simulink model "ACC_ISO_test_001_cs"  (Simulink 7.6)
settings: Solver=ode5  SolverMode=SingleTasking  StartTime=0.0  StopTime=inf  FixedStep=1/100  RelTol=1e-3
PreLoadFcn:
  | check_NUTS_defined;
  | 
  | assignin('base',['model_closed_' bdroot],false);addpath('../includes_ACC');
InitFcn:
  | PreScanExperimentInitFcn(bdroot)
StopFcn:
  | PreScanExperimentStopFcn(bdroot)
undefined symbols (not defined in the file): DiscIntNeverNeededParam, x_ini_VRML, y_ini_VRML, z_ini_VRML
libraries: simulink x26, PreScanSimulinkLibrary x16, simulink_extras x9, PreScanUsefulBlocks x6, simulink_need_slupdate x1
(part 4 of 9)

== system ACC_ISO_test_001_cs/VISUWheels_Mazda_RX8_1 ==
  Wheels : Inport
  Demux : Demux  Outputs=[3 3 3 3 3 3 3 3]
  Saturation{,2,4,6} (4 alike) : Saturate  UpperLimit=[0.2 0.2 0.5]  LowerLimit=[-0.2 -0.2 -0.5]
  Saturation{1,3,5,8} (4 alike) : Saturate  UpperLimit=[30 inf 30]  LowerLimit=[-30 -inf -30]
  conv_RotWheelFL : Subsystem
  conv_RotWheelFR : Subsystem
  conv_RotWheelRL : Subsystem
  conv_RotWheelRR : Subsystem
  conv_TransWheelFL : Subsystem  mask(Translation node configuration){tp=Front-Left Wheel, gains=off, Gain_xISO=1, Gain_yISO=1, Gain_zISO=1}
      mask prompts: tp "Type"; gains "Edit scaling factors?"; Gain_xISO "Scaling factor in x-direction (ISO-convention)"; Gain_yISO "Scaling factor in y-direction (ISO-convention)"; Gain_zISO "Scaling factor in z-direction (ISO-convention)"
      mask init:
      | Visu_ini_param('Mazda_RX8',tp);
      mask StyleString: popup(Front-Left Wheel|Front-Right Wheel|Rear-Left Wheel|Rear-Right Wheel|Left Seat|Right Seat),checkbox,edit,edit,edit
      mask CallbackString:
      | |if strcmp(get_param(gcb, 'gains'),'on')
      |     set_param(gcb,'MaskVisibilities',{'on','on','on','on','on'})
      | else
      |     set_param(gcb,'MaskVisibilities',{'on','on','off','off','off'})
      | end|||
  conv_TransWheelFR : Subsystem  mask(Translation node configuration){tp=Front-Right Wheel, gains=off, Gain_xISO=1, Gain_yISO=1, Gain_zISO=1}
      mask prompts: tp "Type"; gains "Edit scaling factors?"; Gain_xISO "Scaling factor in x-direction (ISO-convention)"; Gain_yISO "Scaling factor in y-direction (ISO-convention)"; Gain_zISO "Scaling factor in z-direction (ISO-convention)"
      mask init:
      | Visu_ini_param('Mazda_RX8',tp);
      mask StyleString: popup(Front-Left Wheel|Front-Right Wheel|Rear-Left Wheel|Rear-Right Wheel|Left Seat|Right Seat),checkbox,edit,edit,edit
      mask CallbackString:
      | |if strcmp(get_param(gcb, 'gains'),'on')
      |     set_param(gcb,'MaskVisibilities',{'on','on','on','on','on'})
      | else
      |     set_param(gcb,'MaskVisibilities',{'on','on','off','off','off'})
      | end|||
  conv_TransWheelRL : Subsystem  mask(Translation node configuration){tp=Rear-Left Wheel, gains=off, Gain_xISO=1, Gain_yISO=1, Gain_zISO=1}
      mask prompts: tp "Type"; gains "Edit scaling factors?"; Gain_xISO "Scaling factor in x-direction (ISO-convention)"; Gain_yISO "Scaling factor in y-direction (ISO-convention)"; Gain_zISO "Scaling factor in z-direction (ISO-convention)"
      mask init:
      | Visu_ini_param('Mazda_RX8',tp);
      mask StyleString: popup(Front-Left Wheel|Front-Right Wheel|Rear-Left Wheel|Rear-Right Wheel|Left Seat|Right Seat),checkbox,edit,edit,edit
      mask CallbackString:
      | |if strcmp(get_param(gcb, 'gains'),'on')
      |     set_param(gcb,'MaskVisibilities',{'on','on','on','on','on'})
      | else
      |     set_param(gcb,'MaskVisibilities',{'on','on','off','off','off'})
      | end|||
  conv_TransWheelRR : Subsystem  mask(Translation node configuration){tp=Rear-Right Wheel, gains=off, Gain_xISO=1, Gain_yISO=1, Gain_zISO=1}
      mask prompts: tp "Type"; gains "Edit scaling factors?"; Gain_xISO "Scaling factor in x-direction (ISO-convention)"; Gain_yISO "Scaling factor in y-direction (ISO-convention)"; Gain_zISO "Scaling factor in z-direction (ISO-convention)"
      mask init:
      | Visu_ini_param('Mazda_RX8',tp);
      mask StyleString: popup(Front-Left Wheel|Front-Right Wheel|Rear-Left Wheel|Rear-Right Wheel|Left Seat|Right Seat),checkbox,edit,edit,edit
      mask CallbackString:
      | |if strcmp(get_param(gcb, 'gains'),'on')
      |     set_param(gcb,'MaskVisibilities',{'on','on','on','on','on'})
      | else
      |     set_param(gcb,'MaskVisibilities',{'on','on','off','off','off'})
      | end|||
  visu_RotWheelFL : Subsystem  mask(ToSensorWorld){PortName=visu_RotWheelFL_0, PortIndex=504, PortWidth=4, TimeStep=1/100}
      mask prompts: PortName "Port Name [-]"; PortIndex "Index [-]"; PortWidth "Port Dimensions [-]"; TimeStep "Upload Period [s]"
      mask help: Sends signal(s) from Simulink to the Sensor World
      mask Help:
      | Sends signal(s) from Simulink to the Sensor World.
      | 
      | - Port Name [-]: specifies the name of the output terminal of the Simulink block.
      | - Index [-]: specifies the start position in the output vector sent to the Sensor World
      | - Port dimensions [-]: specifies the width (number of scalars) of the output port
      | - Upload period [s]: specifies the upload period (in seconds) of the port.
      mask Display: port_label('input', 1, PortName)
  visu_RotWheelFR : Subsystem  mask(ToSensorWorld){PortName=visu_RotWheelFR_0, PortIndex=511, PortWidth=4, TimeStep=1/100}
      mask prompts: PortName "Port Name [-]"; PortIndex "Index [-]"; PortWidth "Port Dimensions [-]"; TimeStep "Upload Period [s]"
      mask help: Sends signal(s) from Simulink to the Sensor World
      mask Help:
      | Sends signal(s) from Simulink to the Sensor World.
      | 
      | - Port Name [-]: specifies the name of the output terminal of the Simulink block.
      | - Index [-]: specifies the start position in the output vector sent to the Sensor World
      | - Port dimensions [-]: specifies the width (number of scalars) of the output port
      | - Upload period [s]: specifies the upload period (in seconds) of the port.
      mask Display: port_label('input', 1, PortName)
  visu_RotWheelRL : Subsystem  mask(ToSensorWorld){PortName=visu_RotWheelRL_0, PortIndex=518, PortWidth=4, TimeStep=1/100}
      mask prompts: PortName "Port Name [-]"; PortIndex "Index [-]"; PortWidth "Port Dimensions [-]"; TimeStep "Upload Period [s]"
      mask help: Sends signal(s) from Simulink to the Sensor World
      mask Help:
      | Sends signal(s) from Simulink to the Sensor World.
      | 
      | - Port Name [-]: specifies the name of the output terminal of the Simulink block.
      | - Index [-]: specifies the start position in the output vector sent to the Sensor World
      | - Port dimensions [-]: specifies the width (number of scalars) of the output port
      | - Upload period [s]: specifies the upload period (in seconds) of the port.
      mask Display: port_label('input', 1, PortName)
  visu_RotWheelRR : Subsystem  mask(ToSensorWorld){PortName=visu_RotWheelRR_0, PortIndex=525, PortWidth=4, TimeStep=1/100}
      mask prompts: PortName "Port Name [-]"; PortIndex "Index [-]"; PortWidth "Port Dimensions [-]"; TimeStep "Upload Period [s]"
      mask help: Sends signal(s) from Simulink to the Sensor World
      mask Help:
      | Sends signal(s) from Simulink to the Sensor World.
      | 
      | - Port Name [-]: specifies the name of the output terminal of the Simulink block.
      | - Index [-]: specifies the start position in the output vector sent to the Sensor World
      | - Port dimensions [-]: specifies the width (number of scalars) of the output port
      | - Upload period [s]: specifies the upload period (in seconds) of the port.
      mask Display: port_label('input', 1, PortName)
  visu_TransWheelFL : Subsystem  mask(ToSensorWorld){PortName=visu_TransWheelFL_0, PortIndex=501, PortWidth=3, TimeStep=1/100}
      mask prompts: PortName "Port Name [-]"; PortIndex "Index [-]"; PortWidth "Port Dimensions [-]"; TimeStep "Upload Period [s]"
      mask help: Sends signal(s) from Simulink to the Sensor World
      mask Help:
      | Sends signal(s) from Simulink to the Sensor World.
      | 
      | - Port Name [-]: specifies the name of the output terminal of the Simulink block.
      | - Index [-]: specifies the start position in the output vector sent to the Sensor World
      | - Port dimensions [-]: specifies the width (number of scalars) of the output port
      | - Upload period [s]: specifies the upload period (in seconds) of the port.
      mask Display: port_label('input', 1, PortName)
  visu_TransWheelFR : Subsystem  mask(ToSensorWorld){PortName=visu_TransWheelFR_0, PortIndex=508, PortWidth=3, TimeStep=1/100}
      mask prompts: PortName "Port Name [-]"; PortIndex "Index [-]"; PortWidth "Port Dimensions [-]"; TimeStep "Upload Period [s]"
      mask help: Sends signal(s) from Simulink to the Sensor World
      mask Help:
      | Sends signal(s) from Simulink to the Sensor World.
      | 
      | - Port Name [-]: specifies the name of the output terminal of the Simulink block.
      | - Index [-]: specifies the start position in the output vector sent to the Sensor World
      | - Port dimensions [-]: specifies the width (number of scalars) of the output port
      | - Upload period [s]: specifies the upload period (in seconds) of the port.
      mask Display: port_label('input', 1, PortName)
  visu_TransWheelRL : Subsystem  mask(ToSensorWorld){PortName=visu_TransWheelRL_0, PortIndex=515, PortWidth=3, TimeStep=1/100}
      mask prompts: PortName "Port Name [-]"; PortIndex "Index [-]"; PortWidth "Port Dimensions [-]"; TimeStep "Upload Period [s]"
      mask help: Sends signal(s) from Simulink to the Sensor World
      mask Help:
      | Sends signal(s) from Simulink to the Sensor World.
      | 
      | - Port Name [-]: specifies the name of the output terminal of the Simulink block.
      | - Index [-]: specifies the start position in the output vector sent to the Sensor World
      | - Port dimensions [-]: specifies the width (number of scalars) of the output port
      | - Upload period [s]: specifies the upload period (in seconds) of the port.
      mask Display: port_label('input', 1, PortName)
  visu_TransWheelRR : Subsystem  mask(ToSensorWorld){PortName=visu_TransWheelRR_0, PortIndex=522, PortWidth=3, TimeStep=1/100}
      mask prompts: PortName "Port Name [-]"; PortIndex "Index [-]"; PortWidth "Port Dimensions [-]"; TimeStep "Upload Period [s]"
      mask help: Sends signal(s) from Simulink to the Sensor World
      mask Help:
      | Sends signal(s) from Simulink to the Sensor World.
      | 
      | - Port Name [-]: specifies the name of the output terminal of the Simulink block.
      | - Index [-]: specifies the start position in the output vector sent to the Sensor World
      | - Port dimensions [-]: specifies the width (number of scalars) of the output port
      | - Upload period [s]: specifies the upload period (in seconds) of the port.
      mask Display: port_label('input', 1, PortName)
  wires:
  conv_RotWheelRR/1(QuaternionVisu [rad]) -> visu_RotWheelRR/1(Y)
  conv_TransWheelRR/1(transVisu [m]) -> visu_TransWheelRR/1(Y)
  conv_RotWheelRL/1(QuaternionVisu [rad]) -> visu_RotWheelRL/1(Y)
  conv_TransWheelRL/1(transVisu [m]) -> visu_TransWheelRL/1(Y)
  conv_RotWheelFR/1(QuaternionVisu [rad]) -> visu_RotWheelFR/1(Y)
  conv_TransWheelFR/1(transVisu [m]) -> visu_TransWheelFR/1(Y)
  conv_RotWheelFL/1(QuaternionVisu [rad]) -> visu_RotWheelFL/1(Y)
  conv_TransWheelFL/1(transVisu [m]) -> visu_TransWheelFL/1(Y)
  Demux/8 -> Saturation5/1
  Demux/7 -> Saturation6/1
  Demux/6 -> Saturation3/1
  Demux/5 -> Saturation4/1
  Demux/4 -> Saturation1/1
  Demux/3 -> Saturation2/1
  Demux/2 -> Saturation8/1
  Demux/1 -> Saturation/1
  Saturation5/1 -> conv_RotWheelRR/1(BryantISO [deg])
  Saturation6/1 -> conv_TransWheelRR/1(transISO [m])
  Saturation3/1 -> conv_RotWheelRL/1(BryantISO [deg])
  Saturation4/1 -> conv_TransWheelRL/1(transISO [m])
  Saturation1/1 -> conv_RotWheelFR/1(BryantISO [deg])
  Saturation2/1 -> conv_TransWheelFR/1(transISO [m])
  Saturation8/1 -> conv_RotWheelFL/1(BryantISO [deg])
  Saturation/1 -> conv_TransWheelFL/1(transISO [m])
  Wheels/1 -> Demux/1  "wheels"

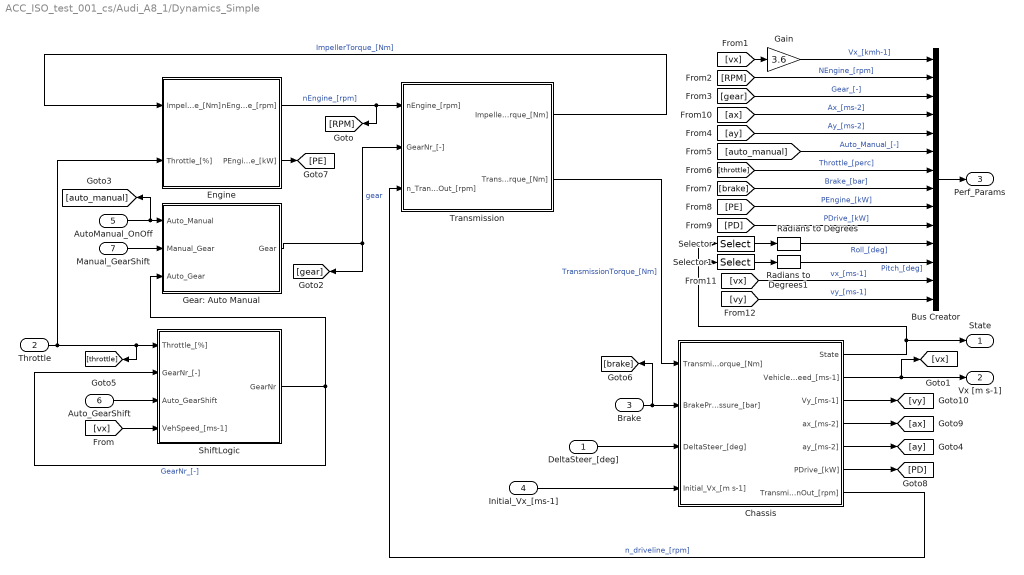
== system ACC_ISO_test_001_cs/Audi_A8_1/Dynamics_Simple ==
  DeltaSteer_[deg] : Inport
  Throttle : Inport  Port=2
  Brake : Inport  Port=3
  Initial_Vx_[ms-1] : Inport  Port=4
  AutoManual_OnOff : Inport  Port=5
  Auto_GearShift : Inport  Port=6
  Manual_GearShift : Inport  Port=7
  Bus Creator : BusCreator  Inputs=14
  Chassis : Subsystem
      mask Display: image(imread('Chassis.png'));
  Engine : Subsystem
      mask Display: image(imread('Engine.png'));
  Gain : Gain  Gain=3.6
  Gear: Auto Manual : Subsystem
  Radians to Degrees : simulink_extras/Transformations/Radians to Degrees  SystemSampleTime=-1
  Radians to Degrees1 : simulink_extras/Transformations/Radians to Degrees  SystemSampleTime=-1
  Selector : Selector  InputPortWidth=9  IndexOptions=Index vector (dialog)  Indices=7  OutputSizes=1
  Selector1 : Selector  InputPortWidth=9  IndexOptions=Index vector (dialog)  Indices=8  OutputSizes=1
  ShiftLogic : Subsystem
      mask Display: image(imread('Gearshift.png'));
  Transmission : Subsystem
      mask Display: image(imread('Transmission.png'));
  State : Outport
  Vx [m s-1] : Outport  Port=2
  Perf_Params : Outport  Port=3
  wires:
  [vy] -> Bus Creator/14  "vy_[ms-1]"
  [vx] -> Bus Creator/13  "vx_[ms-1]"
  Chassis/7(TransmissionOut_[rpm]) -> Transmission/3(n_TransmissionOut_[rpm])  "n_driveline_[rpm]"
  Chassis/6(PDrive_[kW]) -> [PD]
  Chassis/5(ay_[ms-2]) -> [ay]
  Chassis/4(ax_[ms-2]) -> [ax]
  Chassis/3(Vy_[ms-1]) -> [vy]
  [vx] -> ShiftLogic/4(VehSpeed_[ms-1])
  Gear: Auto Manual/1(Gear) -> Transmission/2(GearNr_[-]), [gear]  "gear"
  Manual_GearShift/1 -> Gear: Auto Manual/2(Manual_Gear)
  AutoManual_OnOff/1 -> Gear: Auto Manual/1(Auto_Manual), [auto_manual]
  Chassis/2(VehicleSpeed_[ms-1]) -> [vx], Vx [m s-1]/1
  Auto_GearShift/1 -> ShiftLogic/3(Auto_GearShift)
  Throttle/1 -> Engine/2(Throttle_[%]), ShiftLogic/1(Throttle_[%]), [throttle]
  Initial_Vx_[ms-1]/1 -> Chassis/4(Initial_Vx_[m s-1])
  DeltaSteer_[deg]/1 -> Chassis/3(DeltaSteer_[deg])
  Chassis/1(State) -> State/1, Selector/1, Selector1/1
  Brake/1 -> [brake], Chassis/2(BrakePressure_[bar])
  Engine/1(nEngine_[rpm]) -> [RPM], Transmission/1(nEngine_[rpm])  "nEngine_[rpm]"
  ShiftLogic/1(GearNr) -> Gear: Auto Manual/3(Auto_Gear), ShiftLogic/2(GearNr_[-])  "GearNr_[-]"
  Transmission/2(TransmissionTorque_[Nm]) -> Chassis/1(TransmissionTorque_[Nm])  "TransmissionTorque_[Nm]"
  Transmission/1(ImpellerTorque_[Nm]) -> Engine/1(ImpellerTorque_[Nm])  "ImpellerTorque_[Nm]"
  Gain/1 -> Bus Creator/1  "Vx_[kmh-1]"
  [RPM] -> Bus Creator/2  "NEngine_[rpm]"
  [gear] -> Bus Creator/3  "Gear_[-]"
  [ay] -> Bus Creator/5  "Ay_[ms-2]"
  [auto_manual] -> Bus Creator/6  "Auto_Manual_[-]"
  [throttle] -> Bus Creator/7  "Throttle_[perc]"
  [brake] -> Bus Creator/8  "Brake_[bar]"
  Engine/2(PEngine_[kW]) -> [PE]
  Bus Creator/1 -> Perf_Params/1
  [PE] -> Bus Creator/9  "PEngine_[kW]"
  Radians to Degrees/1 -> Bus Creator/11  "Roll_[deg]"
  Radians to Degrees1/1 -> Bus Creator/12  "Pitch_[deg]"
  [PD] -> Bus Creator/10  "PDrive_[kW]"
  Selector/1 -> Radians to Degrees/1
  Selector1/1 -> Radians to Degrees1/1
  [vx] -> Gain/1
  [ax] -> Bus Creator/4  "Ax_[ms-2]"

== system ACC_ISO_test_001_cs/Audi_A8_1/PathFollower_1 ==
  TrajOffset_x,y,Y [m,m,deg] : Inport
  ActorOffset_Left(+) / Right(-) [m] : Inport  Port=2
  position x,y,Y [m,m,deg] : Inport  Port=3
  Initial Velocity [m/s] : Inport  Port=4
  Desired Velocity [m/s] : Inport  Port=5
  velocity [m/s] : Inport  Port=6
  CTRL REFERENCES : Subsystem
  Calculate shifted p0 wrt COG : Subsystem
  DELTA CTRL : Subsystem
  Demux : Demux  Outputs=3
  Gain : Gain  Gain=1*pi/180
  Goto Tag Visibility : GotoTagVisibility  GotoTag=PreviewDistance
  Goto Tag Visibility1 : GotoTagVisibility  GotoTag=v_actual
  Memory1 : Memory
  Memory2 : Memory
  Memory3 : Memory
  Mux : Mux  Inputs=3
  Preview distance  velocity dependent : Lookup  InputValues=[0 20 30 40 50 60 70 80 90 100 120]  Table=[1 1 2 3 4 5 6 7 10 13.33 20]
  THROTTLE CTRL : Subsystem
  sign1 : Gain  Gain=3.6
  delta_steerwheel [deg] : Outport
  throttle [%] : Outport  Port=2
  brake pressure [bar] : Outport  Port=3
  v0 [m/s] : Outport  Port=4
  Auto_GearShift : Outport  Port=5
  Actor/Traj_distance [m] : Outport  Port=6
  Actor/Traj_angle [deg] : Outport  Port=7
  tag scope: PreviewDistance=scoped, v_actual=scoped
  wires:
  Memory3/1 -> CTRL REFERENCES/4(ActorOffset_Left(+) / Right(-)_[m])
  THROTTLE CTRL/4(Auto_GearShift) -> Auto_GearShift/1
  THROTTLE CTRL/2(brake pressure [bar]) -> brake pressure [bar]/1
  Memory2/1 -> THROTTLE CTRL/1(v_actual [m/s]), [v_actual]
  Memory1/1 -> DELTA CTRL/1(p0), CTRL REFERENCES/1(Pos x,y,Y [m,m,rad])
  sign1/1 -> Preview distance  velocity dependent/1
  Initial Velocity [m/s]/1 -> THROTTLE CTRL/3(Initial Velocity [m/s])
  velocity [m/s]/1 -> Memory2/1
  CTRL REFERENCES/1(pvp  [m,m]) -> DELTA CTRL/2(pvp)
  CTRL REFERENCES/2(pref_pvp [m,m]) -> DELTA CTRL/3(pref_pvp)
  Gain/1 -> Mux/3
  DELTA CTRL/1(delta_steerwheel [deg]) -> delta_steerwheel [deg]/1
  Mux/1 -> CTRL REFERENCES/3(TrajOffset [m,m,rad])
  CTRL REFERENCES/3(pref_0 [m,m]) -> DELTA CTRL/4(pref0)
  THROTTLE CTRL/3(v0 [m/s]) -> v0 [m/s]/1
  THROTTLE CTRL/1(throttle [%]) -> throttle [%]/1
  [v_actual] -> sign1/1
  Preview distance  velocity dependent/1 -> [PreviewDistance], CTRL REFERENCES/2(Position Preview Distance [m])
  Desired Velocity [m/s]/1 -> THROTTLE CTRL/2(Desired Velocity [m/s])
  ActorOffset_Left(+) / Right(-) [m]/1 -> Memory3/1
  Demux/1 -> Mux/1
  Demux/2 -> Mux/2
  Demux/3 -> Gain/1
  TrajOffset_x,y,Y [m,m,deg]/1 -> Demux/1
  Calculate shifted p0 wrt COG/1(position x,y,Y [m,m,rad]) -> Memory1/1
  position x,y,Y [m,m,deg]/1 -> Calculate shifted p0 wrt COG/1(position x,y,Y [m,m,deg])
  CTRL REFERENCES/4(Actor/Traj_distance [m]) -> Actor/Traj_distance [m]/1
  CTRL REFERENCES/5(Actor/Traj_angle [deg]) -> Actor/Traj_angle [deg]/1

== system ACC_ISO_test_001_cs/Audi_A8_1/SELF_Demux ==
  SELF : Inport
  Demux1 : Demux  Outputs=3
  Demux2 : Demux  Outputs=3
  Demux3 : Demux  Outputs=[3 3 1 1]
  Demux4 : Demux  Outputs=3
  Gain : Gain  Gain=180/pi
  Gain1 : Gain  Gain=180/pi
  Selector : Selector  InputPortWidth=3  IndexOptions=Index vector (dialog)  Indices=[3]  OutputSizes=1
  compas converter : Subsystem
  xyz2GPS : PreScanUsefulBlocks/xyz2GPS  CoordinateCount=1  GPS_base=[0.000000 0.000000 0.000]
  x [m] : Outport
  y [m] : Outport  Port=2
  z [m] : Outport  Port=3
  rotx [deg] : Outport  Port=4
  roty [deg] : Outport  Port=5
  rotz [deg] : Outport  Port=6
  GPS lat [deg] : Outport  Port=7
  GPS long [deg] : Outport  Port=8
  GPS alt [m] : Outport  Port=9
  velocity [m/s] : Outport  Port=10
  heading [deg] : Outport  Port=11
  yaw rate [deg/s] : Outport  Port=12
  wires:
  Demux3/4 -> Gain1/1
  Gain1/1 -> yaw rate [deg/s]/1
  Demux3/3 -> velocity [m/s]/1
  compas converter/1(heading [deg]) -> heading [deg]/1
  xyz2GPS/1 -> Demux4/1
  Demux4/3 -> GPS alt [m]/1
  Demux4/2 -> GPS long [deg]/1
  Demux4/1 -> GPS lat [deg]/1
  Demux3/2 -> Gain/1, Selector/1
  Demux3/1 -> xyz2GPS/1, Demux1/1
  SELF/1 -> Demux3/1
  Demux2/3 -> rotz [deg]/1
  Demux2/2 -> roty [deg]/1
  Demux2/1 -> rotx [deg]/1
  Demux1/3 -> z [m]/1
  Demux1/2 -> y [m]/1
  Demux1/1 -> x [m]/1
  Gain/1 -> Demux2/1
  Selector/1 -> compas converter/1(rotz [rad])

== system ACC_ISO_test_001_cs/Audi_A8_1/TIS_1_StandardCoh_Demux ==
  TIS : Inport
  Bus Creator : BusCreator  Inputs=16
  Bus Selector : BusSelector  OutputSignals=ActiveBeamID[-],Range[m],DopplerVelocity[ms-1],DopplerVelocityX[ms-1],DopplerVelocityY[ms-1],DopplerVelocityZ[ms-1],Theta[deg],Phi[deg],TargetID[-],TargetTypeID[-],DopplerVelocityTranslationX[ms-1],DopplerVelocityTranslationY[ms-1],DopplerVelocityTranslationZ[ms-1],DopplerVelocityRotationX[ms-1],DopplerVelocityRotationY[ms-1],DopplerVelocityRotationZ[ms-1]
  ScannerSensorLegacyBusConversion : PreScanUsefulBlocks/ScannerSensorLegacyBusConversion  SystemSampleTime=-1  MAXMESSAGES=MAXMESSAGES
  Out1 : Outport
  Out2 : Outport  Port=2
  Out3 : Outport  Port=3
  Out4 : Outport  Port=4
  Out5 : Outport  Port=5
  Out7 : Outport  Port=6
  Out6 : Outport  Port=7
  wires:
  Bus Selector/16 -> Bus Creator/16  "<DopplerVelocityRotationZ[ms-1]>"
  Bus Selector/15 -> Bus Creator/15  "<DopplerVelocityRotationY[ms-1]>"
  Bus Selector/14 -> Bus Creator/14  "<DopplerVelocityRotationX[ms-1]>"
  Bus Selector/13 -> Bus Creator/13  "<DopplerVelocityTranslationZ[ms-1]>"
  Bus Selector/12 -> Bus Creator/12  "<DopplerVelocityTranslationY[ms-1]>"
  Bus Selector/11 -> Bus Creator/11  "<DopplerVelocityTranslationX[ms-1]>"
  ScannerSensorLegacyBusConversion/1 -> Bus Selector/1
  TIS/1 -> ScannerSensorLegacyBusConversion/1
  Bus Creator/1 -> Out6/1
  Bus Selector/10 -> Bus Creator/10  "<TargetTypeID[-]>"
  Bus Selector/9 -> Out7/1, Bus Creator/9  "<TargetID[-]>"
  Bus Selector/1 -> Out1/1, Bus Creator/1  "<ActiveBeamID[-]>"
  Bus Selector/2 -> Out2/1, Bus Creator/2  "<Range[m]>"
  Bus Selector/7 -> Out4/1, Bus Creator/7  "<Theta[deg]>"
  Bus Selector/8 -> Bus Creator/8, Out5/1  "<Phi[deg]>"
  Bus Selector/3 -> Bus Creator/3, Out3/1  "<DopplerVelocity[ms-1]>"
  Bus Selector/4 -> Bus Creator/4  "<DopplerVelocityX[ms-1]>"
  Bus Selector/5 -> Bus Creator/5  "<DopplerVelocityY[ms-1]>"
  Bus Selector/6 -> Bus Creator/6  "<DopplerVelocityZ[ms-1]>"

== system ACC_ISO_test_001_cs/Audi_A8_1/TIS_2_StandardCoh_Demux ==
  TIS : Inport
  Bus Creator : BusCreator  Inputs=16
  Bus Selector : BusSelector  OutputSignals=ActiveBeamID[-],Range[m],DopplerVelocity[ms-1],DopplerVelocityX[ms-1],DopplerVelocityY[ms-1],DopplerVelocityZ[ms-1],Theta[deg],Phi[deg],TargetID[-],TargetTypeID[-],DopplerVelocityTranslationX[ms-1],DopplerVelocityTranslationY[ms-1],DopplerVelocityTranslationZ[ms-1],DopplerVelocityRotationX[ms-1],DopplerVelocityRotationY[ms-1],DopplerVelocityRotationZ[ms-1]
  ScannerSensorLegacyBusConversion : PreScanUsefulBlocks/ScannerSensorLegacyBusConversion  SystemSampleTime=-1  MAXMESSAGES=MAXMESSAGES
  Out1 : Outport
  Out2 : Outport  Port=2
  Out3 : Outport  Port=3
  Out4 : Outport  Port=4
  Out5 : Outport  Port=5
  Out7 : Outport  Port=6
  Out6 : Outport  Port=7
  wires:
  Bus Selector/16 -> Bus Creator/16  "<DopplerVelocityRotationZ[ms-1]>"
  Bus Selector/15 -> Bus Creator/15  "<DopplerVelocityRotationY[ms-1]>"
  Bus Selector/14 -> Bus Creator/14  "<DopplerVelocityRotationX[ms-1]>"
  Bus Selector/13 -> Bus Creator/13  "<DopplerVelocityTranslationZ[ms-1]>"
  Bus Selector/12 -> Bus Creator/12  "<DopplerVelocityTranslationY[ms-1]>"
  Bus Selector/11 -> Bus Creator/11  "<DopplerVelocityTranslationX[ms-1]>"
  ScannerSensorLegacyBusConversion/1 -> Bus Selector/1
  TIS/1 -> ScannerSensorLegacyBusConversion/1
  Bus Creator/1 -> Out6/1
  Bus Selector/10 -> Bus Creator/10  "<TargetTypeID[-]>"
  Bus Selector/9 -> Out7/1, Bus Creator/9  "<TargetID[-]>"
  Bus Selector/1 -> Out1/1, Bus Creator/1  "<ActiveBeamID[-]>"
  Bus Selector/2 -> Out2/1, Bus Creator/2  "<Range[m]>"
  Bus Selector/7 -> Out4/1, Bus Creator/7  "<Theta[deg]>"
  Bus Selector/8 -> Bus Creator/8, Out5/1  "<Phi[deg]>"
  Bus Selector/3 -> Bus Creator/3, Out3/1  "<DopplerVelocity[ms-1]>"
  Bus Selector/4 -> Bus Creator/4  "<DopplerVelocityX[ms-1]>"
  Bus Selector/5 -> Bus Creator/5  "<DopplerVelocityY[ms-1]>"
  Bus Selector/6 -> Bus Creator/6  "<DopplerVelocityZ[ms-1]>"

== system ACC_ISO_test_001_cs/Audi_A8_1/Trajectories ==
  Traj2State1 : Subsystem  Tag=Traj2State
      settings: DeleteFcn=PreScanBlockDeleteFcn;
      mask Type: PreScan Demux Block:
  Trajectory_1 : Subsystem  Tag=Trajectory  mask(PreScan Source Block: Trajectory){FileName='Trajectory_1.mat', TimeStep=1/100}
      mask prompts: TimeStep "Time Step [s]"
      mask help:
      | The Trajectory block contains the trajectories defined in the PreScan Experiment Editor. The output of the trajectory block is the (vehicle) State.
      |
      | For more information, please click Help.
      mask init:
      | [direc,name]=fileparts(get_param(bdroot, 'FileName'));
      | load([direc,'/Trajectories/',FileName])
      | trajectory=trajectory';
      | 
      | traj.time=trajectory(:,1);%[];
      | traj.signals.values=trajectory(:,2:19);
      | traj.dimensions=18;
      | traj.label='';
      | 
      | SampleTime=traj.time(2)-traj.time(1);
      settings: DeleteFcn=PreScanBlockDeleteFcn;
      mask Help: eval('openHelp(312)')
      mask Display: fprintf(FileName)
  Trajectory_1_Offset : Constant  Tag=TrajectoryOffset  Value="[0  0  0  0  0  0]"
  State : Outport  Tag=TrajOutport
  wires:
  Trajectory_1/1(trajectory) -> Traj2State1/1(Traj Org)
  Trajectory_1_Offset/1 -> Traj2State1/2(Offset)
  Traj2State1/1(state) -> State/1

== system ACC_ISO_test_001_cs/Audi_A8_1/VISULightSource_Mux ==
  IndicatorLightsLeft : Inport
  IndicatorLightsRight : Inport  Port=2
  FogLightRearLeft : Inport  Port=3
  FogLightRearRight : Inport  Port=4
  FogLightFrontLeft : Inport  Port=5
  FogLightFrontRight : Inport  Port=6
  MainLightRearLeft : Inport  Port=7
  MainLightRearRight : Inport  Port=8
  MainLightFrontLeft : Inport  Port=9
  MainLightFrontRight : Inport  Port=10
  BrakeLightLeft : Inport  Port=11
  BrakeLightRight : Inport  Port=12
  SubMuxLightSource : Mux  Inputs=12
  Lights : Outport
  wires:
  SubMuxLightSource/1 -> Lights/1
  IndicatorLightsLeft/1 -> SubMuxLightSource/1
  IndicatorLightsRight/1 -> SubMuxLightSource/2
  FogLightRearLeft/1 -> SubMuxLightSource/3
  FogLightRearRight/1 -> SubMuxLightSource/4
  FogLightFrontLeft/1 -> SubMuxLightSource/5
  FogLightFrontRight/1 -> SubMuxLightSource/6
  MainLightRearLeft/1 -> SubMuxLightSource/7
  MainLightRearRight/1 -> SubMuxLightSource/8
  MainLightFrontLeft/1 -> SubMuxLightSource/9
  MainLightFrontRight/1 -> SubMuxLightSource/10
  BrakeLightLeft/1 -> SubMuxLightSource/11
  BrakeLightRight/1 -> SubMuxLightSource/12

== system ACC_ISO_test_001_cs/Audi_A8_1/VISUSteer_Mux ==
  Column [deg] : Inport
  Steer [deg] : Inport  Port=2
  Mux2 : Mux  Inputs=2
  Steer : Outport
  wires:
  Column [deg]/1 -> Mux2/2
  Mux2/1 -> Steer/1
  Steer [deg]/1 -> Mux2/1

== system ACC_ISO_test_001_cs/Audi_A8_1/VISUWheels_Mux ==
  Steer Angle Front [deg] : Inport  SampleTime=TimeStep
  Steer Angle Rear [deg] : Inport  Port=2  SampleTime=TimeStep
  Velocity [m/s] : Inport  Port=3  SampleTime=TimeStep
  zDisp FL [m] : Inport  Port=4  SampleTime=TimeStep
  zDisp FR [m] : Inport  Port=5  SampleTime=TimeStep
  zDisp RL [m] : Inport  Port=6  SampleTime=TimeStep
  zDisp RR [m] : Inport  Port=7  SampleTime=TimeStep
  Constant{,1..3} (4 alike) : Constant  Value=[0 0]  SampleTime=TimeStep
  Constant{4..7} (4 alike) : Constant  Value=0  SampleTime=TimeStep
  Discrete-Time Integrator : DiscreteIntegrator  SampleTime=TimeStep  ICPrevOutput=DiscIntNeverNeededParam  ICPrevScaledInput=DiscIntNeverNeededParam
  Mux{,1..3} (4 alike) : Mux  Inputs=3
  Mux{4,6..8} (4 alike) : Mux  Inputs=[2 1]
  Mux5 : Mux  Inputs=[3 3 3 3 3 3 3 3]
  Radians to Degrees : simulink_extras/Transformations/Radians to Degrees  SystemSampleTime=-1
  omega=V/Rwheel : Gain  Gain=1/0.29
  Wheels : Outport
  wires:
  Mux7/1 -> Mux5/5  "xyz displacement RL [m]"
  Discrete-Time Integrator/1 -> Mux/2, Mux1/2, Mux2/2, Mux3/2  "roty"
  Radians to Degrees/1 -> Discrete-Time Integrator/1
  Constant7/1 -> Mux3/1  "rotx"
  Constant6/1 -> Mux2/1  "rotx"
  Constant5/1 -> Mux1/1  "rotx"
  Constant4/1 -> Mux/1  "rotx"
  Steer Angle Front [deg]/1 -> Mux1/3, Mux/3  "rotz"
  Steer Angle Rear [deg]/1 -> Mux3/3, Mux2/3  "rotz"
  Mux8/1 -> Mux5/7  "xyz displacement RR [m]"
  Mux6/1 -> Mux5/3  "xyz displacement FR [m]"
  Mux4/1 -> Mux5/1  "xyz displacement FL [m]"
  Constant3/1 -> Mux8/1
  Constant2/1 -> Mux7/1
  Constant1/1 -> Mux6/1
  Constant/1 -> Mux4/1
  zDisp RR [m]/1 -> Mux8/2
  zDisp RL [m]/1 -> Mux7/2
  zDisp FR [m]/1 -> Mux6/2
  zDisp FL [m]/1 -> Mux4/2
  Mux5/1 -> Wheels/1
  omega=V/Rwheel/1 -> Radians to Degrees/1  "rotational speed [rad/s]"
  Velocity [m/s]/1 -> omega=V/Rwheel/1
  Mux1/1 -> Mux5/4  "xyz rotation FR [deg]"
  Mux/1 -> Mux5/2  "xyz rotation FL [deg]"
  Mux3/1 -> Mux5/8  "xyz rotation RR [deg]"
  Mux2/1 -> Mux5/6  "xyz rotation RL [deg]"

== system ACC_ISO_test_001_cs/Audi_A8_1/stop sim ==
  x [m] : Inport
  Relational Operator : RelationalOperator  OutDataTypeStr=boolean
  Stop Simulation : Stop
  wires:
  x [m]/1 -> Relational Operator/1
  [forwardX] -> Relational Operator/2
  Relational Operator/1 -> Stop Simulation/1

== system ACC_ISO_test_001_cs/Audi_A8_1/wheel Z disp ==
  rotY [deg] : Inport
  Degrees to Radians : simulink_extras/Transformations/Degrees to Radians  SystemSampleTime=-1
  Demux : Demux
  Gain : Gain  Gain=[a a -b -b]
  Integer Delay : simulink/Discrete/Integer Delay  NumDelays=1  InputProcessing=Inherited  vinit=0.0  samptime=-1
  Trigonometric Function : Trigonometry  Operator=tan
  zDisp FL [m] : Outport
  zDisp FR [m] : Outport  Port=2
  zDisp RL [m] : Outport  Port=3
  zDisp RR [m] : Outport  Port=4
  wires:
  Demux/4 -> zDisp RR [m]/1
  Demux/3 -> zDisp RL [m]/1
  Demux/2 -> zDisp FR [m]/1
  Demux/1 -> zDisp FL [m]/1
  Gain/1 -> Demux/1
  Trigonometric Function/1 -> Gain/1
  Degrees to Radians/1 -> Trigonometric Function/1
  rotY [deg]/1 -> Integer Delay/1
  Integer Delay/1 -> Degrees to Radians/1

== system ACC_ISO_test_001_cs/BMW_X5_1/SELF_Demux ==
  SELF : Inport
  Demux1 : Demux  Outputs=3
  Demux2 : Demux  Outputs=3
  Demux3 : Demux  Outputs=[3 3 1 1]
  Demux4 : Demux  Outputs=3
  Gain : Gain  Gain=180/pi
  Gain1 : Gain  Gain=180/pi
  Selector : Selector  InputPortWidth=3  IndexOptions=Index vector (dialog)  Indices=[3]  OutputSizes=1
  compas converter : Subsystem
  xyz2GPS : PreScanUsefulBlocks/xyz2GPS  CoordinateCount=1  GPS_base=[0.000000 0.000000 0.000]
  x [m] : Outport
  y [m] : Outport  Port=2
  z [m] : Outport  Port=3
  rotx [deg] : Outport  Port=4
  roty [deg] : Outport  Port=5
  rotz [deg] : Outport  Port=6
  GPS lat [deg] : Outport  Port=7
  GPS long [deg] : Outport  Port=8
  GPS alt [m] : Outport  Port=9
  velocity [m/s] : Outport  Port=10
  heading [deg] : Outport  Port=11
  yaw rate [deg/s] : Outport  Port=12
  wires:
  Demux3/4 -> Gain1/1
  Gain1/1 -> yaw rate [deg/s]/1
  Demux3/3 -> velocity [m/s]/1
  compas converter/1(heading [deg]) -> heading [deg]/1
  xyz2GPS/1 -> Demux4/1
  Demux4/3 -> GPS alt [m]/1
  Demux4/2 -> GPS long [deg]/1
  Demux4/1 -> GPS lat [deg]/1
  Demux3/2 -> Gain/1, Selector/1
  Demux3/1 -> xyz2GPS/1, Demux1/1
  SELF/1 -> Demux3/1
  Demux2/3 -> rotz [deg]/1
  Demux2/2 -> roty [deg]/1
  Demux2/1 -> rotx [deg]/1
  Demux1/3 -> z [m]/1
  Demux1/2 -> y [m]/1
  Demux1/1 -> x [m]/1
  Gain/1 -> Demux2/1
  Selector/1 -> compas converter/1(rotz [rad])

== system ACC_ISO_test_001_cs/BMW_X5_1/Stop_sim ==
  Velocity : Inport
  Clock : Clock
      settings: Decimation=10
  Compare To Zero : simulink/Logic and Bit Operations/Compare To Zero  SystemSampleTime=-1  relop===  LogicOutDataTypeMode=boolean
  Compare To Zero1 : simulink/Logic and Bit Operations/Compare To Zero  SystemSampleTime=-1  relop=~=  LogicOutDataTypeMode=boolean
  Logical Operator : Logic  AllPortsSameDT=off  OutDataTypeStr=boolean
  Stop Simulation : Stop
  wires:
  Clock/1 -> Compare To Zero1/1
  Compare To Zero/1 -> Logical Operator/1
  Compare To Zero1/1 -> Logical Operator/2
  Logical Operator/1 -> Stop Simulation/1
  Velocity/1 -> Compare To Zero/1

== system ACC_ISO_test_001_cs/BMW_X5_1/Trajectories ==
  Traj2State1 : Subsystem  Tag=Traj2State
      settings: DeleteFcn=PreScanBlockDeleteFcn;
      mask Type: PreScan Demux Block:
  Trajectory_2 : Subsystem  Tag=Trajectory  mask(PreScan Source Block: Trajectory){FileName='Trajectory_2.mat', TimeStep=1/100}
      mask prompts: TimeStep "Time Step [s]"
      mask help:
      | The Trajectory block contains the trajectories defined in the PreScan Experiment Editor. The output of the trajectory block is the (vehicle) State.
      |
      | For more information, please click Help.
      mask init: same as ACC_ISO_test_001_cs/Audi_A8_1/Trajectories/Trajectory_1
      settings: DeleteFcn=PreScanBlockDeleteFcn;
      mask Help: eval('openHelp(312)')
      mask Display: fprintf(FileName)
  Trajectory_2_Offset : Constant  Tag=TrajectoryOffset  Value="[0  0  0  0  0  0]"
  State : Outport  Tag=TrajOutport
  wires:
  Trajectory_2/1(trajectory) -> Traj2State1/1(Traj Org)
  Trajectory_2_Offset/1 -> Traj2State1/2(Offset)
  Traj2State1/1(state) -> State/1

== system ACC_ISO_test_001_cs/BMW_X5_1/VISULightSource_Mux ==
  IndicatorLightsLeft : Inport
  IndicatorLightsRight : Inport  Port=2
  FogLightRearLeft : Inport  Port=3
  FogLightRearRight : Inport  Port=4
  FogLightFrontLeft : Inport  Port=5
  FogLightFrontRight : Inport  Port=6
  MainLightRearLeft : Inport  Port=7
  MainLightRearRight : Inport  Port=8
  MainLightFrontLeft : Inport  Port=9
  MainLightFrontRight : Inport  Port=10
  BrakeLightLeft : Inport  Port=11
  BrakeLightRight : Inport  Port=12
  SubMuxLightSource : Mux  Inputs=12
  Lights : Outport
  wires:
  SubMuxLightSource/1 -> Lights/1
  IndicatorLightsLeft/1 -> SubMuxLightSource/1
  IndicatorLightsRight/1 -> SubMuxLightSource/2
  FogLightRearLeft/1 -> SubMuxLightSource/3
  FogLightRearRight/1 -> SubMuxLightSource/4
  FogLightFrontLeft/1 -> SubMuxLightSource/5
  FogLightFrontRight/1 -> SubMuxLightSource/6
  MainLightRearLeft/1 -> SubMuxLightSource/7
  MainLightRearRight/1 -> SubMuxLightSource/8
  MainLightFrontLeft/1 -> SubMuxLightSource/9
  MainLightFrontRight/1 -> SubMuxLightSource/10
  BrakeLightLeft/1 -> SubMuxLightSource/11
  BrakeLightRight/1 -> SubMuxLightSource/12

== system ACC_ISO_test_001_cs/BMW_X5_1/VISUSteer_Mux ==
  Column [deg] : Inport
  Steer [deg] : Inport  Port=2
  Mux2 : Mux  Inputs=2
  Steer : Outport
  wires:
  Column [deg]/1 -> Mux2/2
  Mux2/1 -> Steer/1
  Steer [deg]/1 -> Mux2/1

== system ACC_ISO_test_001_cs/BMW_X5_1/VISUWheels_Mux ==
  Steer Angle Front [deg] : Inport  SampleTime=TimeStep
  Steer Angle Rear [deg] : Inport  Port=2  SampleTime=TimeStep
  Velocity [m/s] : Inport  Port=3  SampleTime=TimeStep
  zDisp FL [m] : Inport  Port=4  SampleTime=TimeStep
  zDisp FR [m] : Inport  Port=5  SampleTime=TimeStep
  zDisp RL [m] : Inport  Port=6  SampleTime=TimeStep
  zDisp RR [m] : Inport  Port=7  SampleTime=TimeStep
  Constant{,1..3} (4 alike) : Constant  Value=[0 0]  SampleTime=TimeStep
  Constant{4..7} (4 alike) : Constant  Value=0  SampleTime=TimeStep
  Discrete-Time Integrator : DiscreteIntegrator  SampleTime=TimeStep  ICPrevOutput=DiscIntNeverNeededParam  ICPrevScaledInput=DiscIntNeverNeededParam
  Mux{,1..3} (4 alike) : Mux  Inputs=3
  Mux{4,6..8} (4 alike) : Mux  Inputs=[2 1]
  Mux5 : Mux  Inputs=[3 3 3 3 3 3 3 3]
  Radians to Degrees : simulink_extras/Transformations/Radians to Degrees  SystemSampleTime=-1
  omega=V/Rwheel : Gain  Gain=1/0.29
  Wheels : Outport
  wires:
  Mux7/1 -> Mux5/5  "xyz displacement RL [m]"
  Discrete-Time Integrator/1 -> Mux/2, Mux1/2, Mux2/2, Mux3/2  "roty"
  Radians to Degrees/1 -> Discrete-Time Integrator/1
  Constant7/1 -> Mux3/1  "rotx"
  Constant6/1 -> Mux2/1  "rotx"
  Constant5/1 -> Mux1/1  "rotx"
  Constant4/1 -> Mux/1  "rotx"
  Steer Angle Front [deg]/1 -> Mux1/3, Mux/3  "rotz"
  Steer Angle Rear [deg]/1 -> Mux3/3, Mux2/3  "rotz"
  Mux8/1 -> Mux5/7  "xyz displacement RR [m]"
  Mux6/1 -> Mux5/3  "xyz displacement FR [m]"
  Mux4/1 -> Mux5/1  "xyz displacement FL [m]"
  Constant3/1 -> Mux8/1
  Constant2/1 -> Mux7/1
  Constant1/1 -> Mux6/1
  Constant/1 -> Mux4/1
  zDisp RR [m]/1 -> Mux8/2
  zDisp RL [m]/1 -> Mux7/2
  zDisp FR [m]/1 -> Mux6/2
  zDisp FL [m]/1 -> Mux4/2
  Mux5/1 -> Wheels/1
  omega=V/Rwheel/1 -> Radians to Degrees/1  "rotational speed [rad/s]"
  Velocity [m/s]/1 -> omega=V/Rwheel/1
  Mux1/1 -> Mux5/4  "xyz rotation FR [deg]"
  Mux/1 -> Mux5/2  "xyz rotation FL [deg]"
  Mux3/1 -> Mux5/8  "xyz rotation RR [deg]"
  Mux2/1 -> Mux5/6  "xyz rotation RL [deg]"

== system ACC_ISO_test_001_cs/Mazda_RX8_1/SELF_Demux ==
  SELF : Inport
  Demux1 : Demux  Outputs=3
  Demux2 : Demux  Outputs=3
  Demux3 : Demux  Outputs=[3 3 1 1]
  Demux4 : Demux  Outputs=3
  Gain : Gain  Gain=180/pi
  Gain1 : Gain  Gain=180/pi
  Selector : Selector  InputPortWidth=3  IndexOptions=Index vector (dialog)  Indices=[3]  OutputSizes=1
  compas converter : Subsystem
  xyz2GPS : PreScanUsefulBlocks/xyz2GPS  CoordinateCount=1  GPS_base=[0.000000 0.000000 0.000]
  x [m] : Outport
  y [m] : Outport  Port=2
  z [m] : Outport  Port=3
  rotx [deg] : Outport  Port=4
  roty [deg] : Outport  Port=5
  rotz [deg] : Outport  Port=6
  GPS lat [deg] : Outport  Port=7
  GPS long [deg] : Outport  Port=8
  GPS alt [m] : Outport  Port=9
  velocity [m/s] : Outport  Port=10
  heading [deg] : Outport  Port=11
  yaw rate [deg/s] : Outport  Port=12
  wires:
  Demux3/4 -> Gain1/1
  Gain1/1 -> yaw rate [deg/s]/1
  Demux3/3 -> velocity [m/s]/1
  compas converter/1(heading [deg]) -> heading [deg]/1
  xyz2GPS/1 -> Demux4/1
  Demux4/3 -> GPS alt [m]/1
  Demux4/2 -> GPS long [deg]/1
  Demux4/1 -> GPS lat [deg]/1
  Demux3/2 -> Gain/1, Selector/1
  Demux3/1 -> xyz2GPS/1, Demux1/1
  SELF/1 -> Demux3/1
  Demux2/3 -> rotz [deg]/1
  Demux2/2 -> roty [deg]/1
  Demux2/1 -> rotx [deg]/1
  Demux1/3 -> z [m]/1
  Demux1/2 -> y [m]/1
  Demux1/1 -> x [m]/1
  Gain/1 -> Demux2/1
  Selector/1 -> compas converter/1(rotz [rad])

== system ACC_ISO_test_001_cs/Mazda_RX8_1/Trajectories ==
  Traj2State1 : Subsystem  Tag=Traj2State
      settings: DeleteFcn=PreScanBlockDeleteFcn;
      mask Type: PreScan Demux Block:
  Trajectory_3 : Subsystem  Tag=Trajectory  mask(PreScan Source Block: Trajectory){FileName='Trajectory_3.mat', TimeStep=1/100}
      mask prompts: TimeStep "Time Step [s]"
      mask help:
      | The Trajectory block contains the trajectories defined in the PreScan Experiment Editor. The output of the trajectory block is the (vehicle) State.
      |
      | For more information, please click Help.
      mask init: same as ACC_ISO_test_001_cs/Audi_A8_1/Trajectories/Trajectory_1
      settings: DeleteFcn=PreScanBlockDeleteFcn;
      mask Help: eval('openHelp(312)')
      mask Display: fprintf(FileName)
  Trajectory_3_Offset : Constant  Tag=TrajectoryOffset  Value="[0  0  0  0  0  0]"
  State : Outport  Tag=TrajOutport
  wires:
  Trajectory_3/1(trajectory) -> Traj2State1/1(Traj Org)
  Trajectory_3_Offset/1 -> Traj2State1/2(Offset)
  Traj2State1/1(state) -> State/1

== system ACC_ISO_test_001_cs/Mazda_RX8_1/VISULightSource_Mux ==
  IndicatorLightsLeft : Inport
  IndicatorLightsRight : Inport  Port=2
  FogLightRearLeft : Inport  Port=3
  FogLightRearRight : Inport  Port=4
  FogLightFrontLeft : Inport  Port=5
  FogLightFrontRight : Inport  Port=6
  MainLightRearLeft : Inport  Port=7
  MainLightRearRight : Inport  Port=8
  MainLightFrontLeft : Inport  Port=9
  MainLightFrontRight : Inport  Port=10
  BrakeLightLeft : Inport  Port=11
  BrakeLightMiddle : Inport  Port=12
  BrakeLightRight : Inport  Port=13
  SubMuxLightSource : Mux  Inputs=13
  Lights : Outport
  wires:
  SubMuxLightSource/1 -> Lights/1
  IndicatorLightsLeft/1 -> SubMuxLightSource/1
  IndicatorLightsRight/1 -> SubMuxLightSource/2
  FogLightRearLeft/1 -> SubMuxLightSource/3
  FogLightRearRight/1 -> SubMuxLightSource/4
  FogLightFrontLeft/1 -> SubMuxLightSource/5
  FogLightFrontRight/1 -> SubMuxLightSource/6
  MainLightRearLeft/1 -> SubMuxLightSource/7
  MainLightRearRight/1 -> SubMuxLightSource/8
  MainLightFrontLeft/1 -> SubMuxLightSource/9
  MainLightFrontRight/1 -> SubMuxLightSource/10
  BrakeLightLeft/1 -> SubMuxLightSource/11
  BrakeLightMiddle/1 -> SubMuxLightSource/12
  BrakeLightRight/1 -> SubMuxLightSource/13

== system ACC_ISO_test_001_cs/Mazda_RX8_1/VISUSteer_Mux ==
  Column [deg] : Inport
  Steer [deg] : Inport  Port=2
  Mux2 : Mux  Inputs=2
  Steer : Outport
  wires:
  Column [deg]/1 -> Mux2/2
  Mux2/1 -> Steer/1
  Steer [deg]/1 -> Mux2/1

== system ACC_ISO_test_001_cs/Mazda_RX8_1/VISUWheels_Mux ==
  Steer Angle Front [deg] : Inport  SampleTime=TimeStep
  Steer Angle Rear [deg] : Inport  Port=2  SampleTime=TimeStep
  Velocity [m/s] : Inport  Port=3  SampleTime=TimeStep
  zDisp FL [m] : Inport  Port=4  SampleTime=TimeStep
  zDisp FR [m] : Inport  Port=5  SampleTime=TimeStep
  zDisp RL [m] : Inport  Port=6  SampleTime=TimeStep
  zDisp RR [m] : Inport  Port=7  SampleTime=TimeStep
  Constant{,1..3} (4 alike) : Constant  Value=[0 0]  SampleTime=TimeStep
  Constant{4..7} (4 alike) : Constant  Value=0  SampleTime=TimeStep
  Discrete-Time Integrator : DiscreteIntegrator  SampleTime=TimeStep  ICPrevOutput=DiscIntNeverNeededParam  ICPrevScaledInput=DiscIntNeverNeededParam
  Mux{,1..3} (4 alike) : Mux  Inputs=3
  Mux{4,6..8} (4 alike) : Mux  Inputs=[2 1]
  Mux5 : Mux  Inputs=[3 3 3 3 3 3 3 3]
  Radians to Degrees : simulink_extras/Transformations/Radians to Degrees  SystemSampleTime=-1
  omega=V/Rwheel : Gain  Gain=1/0.29
  Wheels : Outport
  wires:
  Mux7/1 -> Mux5/5  "xyz displacement RL [m]"
  Discrete-Time Integrator/1 -> Mux/2, Mux1/2, Mux2/2, Mux3/2  "roty"
  Radians to Degrees/1 -> Discrete-Time Integrator/1
  Constant7/1 -> Mux3/1  "rotx"
  Constant6/1 -> Mux2/1  "rotx"
  Constant5/1 -> Mux1/1  "rotx"
  Constant4/1 -> Mux/1  "rotx"
  Steer Angle Front [deg]/1 -> Mux1/3, Mux/3  "rotz"
  Steer Angle Rear [deg]/1 -> Mux3/3, Mux2/3  "rotz"
  Mux8/1 -> Mux5/7  "xyz displacement RR [m]"
  Mux6/1 -> Mux5/3  "xyz displacement FR [m]"
  Mux4/1 -> Mux5/1  "xyz displacement FL [m]"
  Constant3/1 -> Mux8/1
  Constant2/1 -> Mux7/1
  Constant1/1 -> Mux6/1
  Constant/1 -> Mux4/1
  zDisp RR [m]/1 -> Mux8/2
  zDisp RL [m]/1 -> Mux7/2
  zDisp FR [m]/1 -> Mux6/2
  zDisp FL [m]/1 -> Mux4/2
  Mux5/1 -> Wheels/1
  omega=V/Rwheel/1 -> Radians to Degrees/1  "rotational speed [rad/s]"
  Velocity [m/s]/1 -> omega=V/Rwheel/1
  Mux1/1 -> Mux5/4  "xyz rotation FR [deg]"
  Mux/1 -> Mux5/2  "xyz rotation FL [deg]"
  Mux3/1 -> Mux5/8  "xyz rotation RR [deg]"
  Mux2/1 -> Mux5/6  "xyz rotation RL [deg]"

== system ACC_ISO_test_001_cs/STATE_Audi_A8_1/Acceleration ==
  Y : Inport
  Assignment : Assignment  IndexMode=Zero-based  SampleTime=TimeStep  IndexOptions=Starting index (dialog)  Indices=PortIndex  OutputSizes=[1 1]
  Data Store Read : DataStoreRead  DataStoreName=SimCoreActuators  SampleTime=TimeStep
  Data Store Write : DataStoreWrite  DataStoreName=SimCoreActuators
  wires:
  Assignment/1 -> Data Store Write/1
  Data Store Read/1 -> Assignment/1
  Y/1 -> Assignment/2

== system ACC_ISO_test_001_cs/STATE_Audi_A8_1/Position ==
  Y : Inport
  Assignment : Assignment  IndexMode=Zero-based  SampleTime=TimeStep  IndexOptions=Starting index (dialog)  Indices=PortIndex  OutputSizes=[1 1]
  Data Store Read : DataStoreRead  DataStoreName=SimCoreActuators  SampleTime=TimeStep
  Data Store Write : DataStoreWrite  DataStoreName=SimCoreActuators
  wires:
  Y/1 -> Assignment/2
  Data Store Read/1 -> Assignment/1
  Assignment/1 -> Data Store Write/1

== system ACC_ISO_test_001_cs/STATE_Audi_A8_1/RPY ==
  Y : Inport
  Assignment : Assignment  IndexMode=Zero-based  SampleTime=TimeStep  IndexOptions=Starting index (dialog)  Indices=PortIndex  OutputSizes=[1 1]
  Data Store Read : DataStoreRead  DataStoreName=SimCoreActuators  SampleTime=TimeStep
  Data Store Write : DataStoreWrite  DataStoreName=SimCoreActuators
  wires:
  Assignment/1 -> Data Store Write/1
  Data Store Read/1 -> Assignment/1
  Y/1 -> Assignment/2

== system ACC_ISO_test_001_cs/STATE_Audi_A8_1/Velocity ==
  Y : Inport
  Assignment : Assignment  IndexMode=Zero-based  SampleTime=TimeStep  IndexOptions=Starting index (dialog)  Indices=PortIndex  OutputSizes=[1 1]
  Data Store Read : DataStoreRead  DataStoreName=SimCoreActuators  SampleTime=TimeStep
  Data Store Write : DataStoreWrite  DataStoreName=SimCoreActuators
  wires:
  Assignment/1 -> Data Store Write/1
  Data Store Read/1 -> Assignment/1
  Y/1 -> Assignment/2

== system ACC_ISO_test_001_cs/STATE_Audi_A8_1/velRPY ==
  Y : Inport
  Assignment : Assignment  IndexMode=Zero-based  SampleTime=TimeStep  IndexOptions=Starting index (dialog)  Indices=PortIndex  OutputSizes=[1 1]
  Data Store Read : DataStoreRead  DataStoreName=SimCoreActuators  SampleTime=TimeStep
  Data Store Write : DataStoreWrite  DataStoreName=SimCoreActuators
  wires:
  Assignment/1 -> Data Store Write/1
  Data Store Read/1 -> Assignment/1
  Y/1 -> Assignment/2

== system ACC_ISO_test_001_cs/STATE_BMW_X5_1/Acceleration ==
  Y : Inport
  Assignment : Assignment  IndexMode=Zero-based  SampleTime=TimeStep  IndexOptions=Starting index (dialog)  Indices=PortIndex  OutputSizes=[1 1]
  Data Store Read : DataStoreRead  DataStoreName=SimCoreActuators  SampleTime=TimeStep
  Data Store Write : DataStoreWrite  DataStoreName=SimCoreActuators
  wires:
  Assignment/1 -> Data Store Write/1
  Data Store Read/1 -> Assignment/1
  Y/1 -> Assignment/2

== system ACC_ISO_test_001_cs/STATE_BMW_X5_1/Position ==
  Y : Inport
  Assignment : Assignment  IndexMode=Zero-based  SampleTime=TimeStep  IndexOptions=Starting index (dialog)  Indices=PortIndex  OutputSizes=[1 1]
  Data Store Read : DataStoreRead  DataStoreName=SimCoreActuators  SampleTime=TimeStep
  Data Store Write : DataStoreWrite  DataStoreName=SimCoreActuators
  wires:
  Y/1 -> Assignment/2
  Data Store Read/1 -> Assignment/1
  Assignment/1 -> Data Store Write/1

== system ACC_ISO_test_001_cs/STATE_BMW_X5_1/RPY ==
  Y : Inport
  Assignment : Assignment  IndexMode=Zero-based  SampleTime=TimeStep  IndexOptions=Starting index (dialog)  Indices=PortIndex  OutputSizes=[1 1]
  Data Store Read : DataStoreRead  DataStoreName=SimCoreActuators  SampleTime=TimeStep
  Data Store Write : DataStoreWrite  DataStoreName=SimCoreActuators
  wires:
  Assignment/1 -> Data Store Write/1
  Data Store Read/1 -> Assignment/1
  Y/1 -> Assignment/2

== system ACC_ISO_test_001_cs/STATE_BMW_X5_1/Velocity ==
  Y : Inport
  Assignment : Assignment  IndexMode=Zero-based  SampleTime=TimeStep  IndexOptions=Starting index (dialog)  Indices=PortIndex  OutputSizes=[1 1]
  Data Store Read : DataStoreRead  DataStoreName=SimCoreActuators  SampleTime=TimeStep
  Data Store Write : DataStoreWrite  DataStoreName=SimCoreActuators
  wires:
  Assignment/1 -> Data Store Write/1
  Data Store Read/1 -> Assignment/1
  Y/1 -> Assignment/2

== system ACC_ISO_test_001_cs/STATE_BMW_X5_1/velRPY ==
  Y : Inport
  Assignment : Assignment  IndexMode=Zero-based  SampleTime=TimeStep  IndexOptions=Starting index (dialog)  Indices=PortIndex  OutputSizes=[1 1]
  Data Store Read : DataStoreRead  DataStoreName=SimCoreActuators  SampleTime=TimeStep
  Data Store Write : DataStoreWrite  DataStoreName=SimCoreActuators
  wires:
  Assignment/1 -> Data Store Write/1
  Data Store Read/1 -> Assignment/1
  Y/1 -> Assignment/2

== system ACC_ISO_test_001_cs/STATE_Mazda_RX8_1/Acceleration ==
  Y : Inport
  Assignment : Assignment  IndexMode=Zero-based  SampleTime=TimeStep  IndexOptions=Starting index (dialog)  Indices=PortIndex  OutputSizes=[1 1]
  Data Store Read : DataStoreRead  DataStoreName=SimCoreActuators  SampleTime=TimeStep
  Data Store Write : DataStoreWrite  DataStoreName=SimCoreActuators
  wires:
  Assignment/1 -> Data Store Write/1
  Data Store Read/1 -> Assignment/1
  Y/1 -> Assignment/2

== system ACC_ISO_test_001_cs/STATE_Mazda_RX8_1/Position ==
  Y : Inport
  Assignment : Assignment  IndexMode=Zero-based  SampleTime=TimeStep  IndexOptions=Starting index (dialog)  Indices=PortIndex  OutputSizes=[1 1]
  Data Store Read : DataStoreRead  DataStoreName=SimCoreActuators  SampleTime=TimeStep
  Data Store Write : DataStoreWrite  DataStoreName=SimCoreActuators
  wires:
  Y/1 -> Assignment/2
  Data Store Read/1 -> Assignment/1
  Assignment/1 -> Data Store Write/1

== system ACC_ISO_test_001_cs/STATE_Mazda_RX8_1/RPY ==
  Y : Inport
  Assignment : Assignment  IndexMode=Zero-based  SampleTime=TimeStep  IndexOptions=Starting index (dialog)  Indices=PortIndex  OutputSizes=[1 1]
  Data Store Read : DataStoreRead  DataStoreName=SimCoreActuators  SampleTime=TimeStep
  Data Store Write : DataStoreWrite  DataStoreName=SimCoreActuators
  wires:
  Assignment/1 -> Data Store Write/1
  Data Store Read/1 -> Assignment/1
  Y/1 -> Assignment/2

== system ACC_ISO_test_001_cs/STATE_Mazda_RX8_1/Velocity ==
  Y : Inport
  Assignment : Assignment  IndexMode=Zero-based  SampleTime=TimeStep  IndexOptions=Starting index (dialog)  Indices=PortIndex  OutputSizes=[1 1]
  Data Store Read : DataStoreRead  DataStoreName=SimCoreActuators  SampleTime=TimeStep
  Data Store Write : DataStoreWrite  DataStoreName=SimCoreActuators
  wires:
  Assignment/1 -> Data Store Write/1
  Data Store Read/1 -> Assignment/1
  Y/1 -> Assignment/2
